simulink model "ft33_project2"  (R2024a)
settings: Solver=VariableStepAuto  StartTime=0.0  StopTime=10.0  RelTol=1e-3
undefined symbols (not defined in the file or in its folder): ft33_project2_copy, Subsystem16, xc7z020clg484
libraries: hdlBasic x111, vmcUtilities x1
(part 2 of 2)

== system ft33_project2/Subsystem16/Subsystem4 ==
  InA : Inport
  ShiftIn : Inport  Port=2
  Select : Inport  Port=3
  InB : Inport  Port=4
  Reset : Inport  Port=5
  Accumulator : hdlBasic/Accumulator  operation=Add  n_bits=16  overflow=Flag as error  scale=1  rst=on  hasbypass=off  en=off  latency=1  msb_inp=100  msb=100  lsb=-100  use_behavioral_HDL=on  implementation=Fabric  XmcBlockStatus=1  maskContainerNames=group3  block_type=accum  block_config=sysgen:Accum_config  block_width=566  block_height=845
  Delay : hdlBasic/Delay  rst=off  en=off  latency=1  reg_retiming=off  XmcBlockStatus=1  maskContainerNames=group1  block_type=delay  block_config=sysgen:Delay_config
  DelayA : hdlBasic/Register  init=0  rst=off  en=off  XmcBlockStatus=1  maskContainerNames=tabcontainer1  block_type=register  block_config=sysgen:Register_config
  DelayB : hdlBasic/Register  init=0  rst=off  en=off  XmcBlockStatus=1  maskContainerNames=tabcontainer1  block_type=register  block_config=sysgen:Register_config
  Mult : hdlBasic/Mult  precision=User Defined  arith_type="Signed  (2's comp)"  n_bits=16  bin_pt=0  quantization=Truncate  overflow=Wrap  en=off  latency=1  opt_float=off  fp_mult_usage=No Usage  use_behavioral_HDL=off  opt=Speed  use_embedded=on  optimum_pipeline=off  pipeline=on  use_rpm=on  placement_style=Triangular  XmcBlockStatus=1  maskContainerNames=group1  block_type=mult  block_config=sysgen:Mult_config  block_width=598  block_height=876
  Mux : hdlBasic/Mux  inputs=2  en=off  latency=1  precision=Full  arith_type=Unsigned  n_bits=16  bin_pt=14  quantization=Truncate  overflow=Wrap  XmcBlockStatus=1  maskContainerNames=tabcontainer1  block_type=mux  block_config=sysgen:Mux_config
  OutA : Outport
  ShiftOut : Outport  Port=2
  ResetOut : Outport  Port=3
  OutB : Outport  Port=4
  wires:
  Accumulator/1 -> Mux/2
  Mult/1 -> Accumulator/1
  InB/1 -> DelayB/1, Mult/2
  Select/1 -> Mux/1
  ShiftIn/1 -> Mux/3
  Mux/1 -> ShiftOut/1
  Reset/1 -> Delay/1, Accumulator/2
  InA/1 -> Mult/1, DelayA/1
  DelayA/1 -> OutA/1
  DelayB/1 -> OutB/1
  Delay/1 -> ResetOut/1

== system ft33_project2/Subsystem16/Subsystem5 ==
  InA : Inport
  ShiftIn : Inport  Port=2
  Select : Inport  Port=3
  InB : Inport  Port=4
  Reset : Inport  Port=5
  Accumulator : hdlBasic/Accumulator  operation=Add  n_bits=16  overflow=Flag as error  scale=1  rst=on  hasbypass=off  en=off  latency=1  msb_inp=100  msb=100  lsb=-100  use_behavioral_HDL=on  implementation=Fabric  XmcBlockStatus=1  maskContainerNames=group3  block_type=accum  block_config=sysgen:Accum_config  block_width=566  block_height=845
  Delay : hdlBasic/Delay  rst=off  en=off  latency=1  reg_retiming=off  XmcBlockStatus=1  maskContainerNames=group1  block_type=delay  block_config=sysgen:Delay_config
  DelayA : hdlBasic/Register  init=0  rst=off  en=off  XmcBlockStatus=1  maskContainerNames=tabcontainer1  block_type=register  block_config=sysgen:Register_config
  DelayB : hdlBasic/Register  init=0  rst=off  en=off  XmcBlockStatus=1  maskContainerNames=tabcontainer1  block_type=register  block_config=sysgen:Register_config
  Mult : hdlBasic/Mult  precision=User Defined  arith_type="Signed  (2's comp)"  n_bits=16  bin_pt=0  quantization=Truncate  overflow=Wrap  en=off  latency=1  opt_float=off  fp_mult_usage=No Usage  use_behavioral_HDL=off  opt=Speed  use_embedded=on  optimum_pipeline=off  pipeline=on  use_rpm=on  placement_style=Triangular  XmcBlockStatus=1  maskContainerNames=group1  block_type=mult  block_config=sysgen:Mult_config  block_width=598  block_height=876
  Mux : hdlBasic/Mux  inputs=2  en=off  latency=1  precision=Full  arith_type=Unsigned  n_bits=16  bin_pt=14  quantization=Truncate  overflow=Wrap  XmcBlockStatus=1  maskContainerNames=tabcontainer1  block_type=mux  block_config=sysgen:Mux_config
  OutA : Outport
  ShiftOut : Outport  Port=2
  ResetOut : Outport  Port=3
  OutB : Outport  Port=4
  wires:
  Accumulator/1 -> Mux/2
  Mult/1 -> Accumulator/1
  InB/1 -> DelayB/1, Mult/2
  Select/1 -> Mux/1
  ShiftIn/1 -> Mux/3
  Mux/1 -> ShiftOut/1
  Reset/1 -> Delay/1, Accumulator/2
  InA/1 -> Mult/1, DelayA/1
  DelayA/1 -> OutA/1
  DelayB/1 -> OutB/1
  Delay/1 -> ResetOut/1

== system ft33_project2/Subsystem16/Subsystem6 ==
  InA : Inport
  ShiftIn : Inport  Port=2
  ResetIn : Inport  Port=3
  Select : Inport  Port=4
  InB : Inport  Port=5
  Accumulator : hdlBasic/Accumulator  operation=Add  n_bits=16  overflow=Flag as error  scale=1  rst=on  hasbypass=off  en=off  latency=1  msb_inp=100  msb=100  lsb=-100  use_behavioral_HDL=on  implementation=Fabric  XmcBlockStatus=1  maskContainerNames=group3  block_type=accum  block_config=sysgen:Accum_config  block_width=566  block_height=845
  Delay : hdlBasic/Delay  rst=off  en=off  latency=1  reg_retiming=off  XmcBlockStatus=1  maskContainerNames=group1  block_type=delay  block_config=sysgen:Delay_config
  DelayA : hdlBasic/Register  init=0  rst=off  en=off  XmcBlockStatus=1  maskContainerNames=tabcontainer1  block_type=register  block_config=sysgen:Register_config
  DelayB : hdlBasic/Register  init=0  rst=off  en=off  XmcBlockStatus=1  maskContainerNames=tabcontainer1  block_type=register  block_config=sysgen:Register_config
  Mult : hdlBasic/Mult  precision=User Defined  arith_type="Signed  (2's comp)"  n_bits=16  bin_pt=0  quantization=Truncate  overflow=Wrap  en=off  latency=1  opt_float=off  fp_mult_usage=No Usage  use_behavioral_HDL=off  opt=Speed  use_embedded=on  optimum_pipeline=off  pipeline=on  use_rpm=on  placement_style=Triangular  XmcBlockStatus=1  maskContainerNames=group1  block_type=mult  block_config=sysgen:Mult_config  block_width=598  block_height=876
  Mux : hdlBasic/Mux  inputs=2  en=off  latency=1  precision=Full  arith_type=Unsigned  n_bits=16  bin_pt=14  quantization=Truncate  overflow=Wrap  XmcBlockStatus=1  maskContainerNames=tabcontainer1  block_type=mux  block_config=sysgen:Mux_config
  OutA : Outport
  ShiftOut : Outport  Port=2
  ResetOut : Outport  Port=3
  OutB : Outport  Port=4
  wires:
  Accumulator/1 -> Mux/2
  Mult/1 -> Accumulator/1
  InB/1 -> DelayB/1, Mult/2
  Select/1 -> Mux/1
  ShiftIn/1 -> Mux/3
  Mux/1 -> ShiftOut/1
  ResetIn/1 -> Delay/1, Accumulator/2
  InA/1 -> Mult/1, DelayA/1
  DelayA/1 -> OutA/1
  DelayB/1 -> OutB/1
  Delay/1 -> ResetOut/1

== system ft33_project2/Subsystem16/Subsystem7 ==
  InA : Inport
  ShiftIn : Inport  Port=2
  ResetIn : Inport  Port=3
  Select : Inport  Port=4
  InB : Inport  Port=5
  Accumulator : hdlBasic/Accumulator  operation=Add  n_bits=16  overflow=Flag as error  scale=1  rst=on  hasbypass=off  en=off  latency=1  msb_inp=100  msb=100  lsb=-100  use_behavioral_HDL=on  implementation=Fabric  XmcBlockStatus=1  maskContainerNames=group3  block_type=accum  block_config=sysgen:Accum_config  block_width=566  block_height=845
  Delay : hdlBasic/Delay  rst=off  en=off  latency=1  reg_retiming=off  XmcBlockStatus=1  maskContainerNames=group1  block_type=delay  block_config=sysgen:Delay_config
  DelayA : hdlBasic/Register  init=0  rst=off  en=off  XmcBlockStatus=1  maskContainerNames=tabcontainer1  block_type=register  block_config=sysgen:Register_config
  DelayB : hdlBasic/Register  init=0  rst=off  en=off  XmcBlockStatus=1  maskContainerNames=tabcontainer1  block_type=register  block_config=sysgen:Register_config
  Mult : hdlBasic/Mult  precision=User Defined  arith_type="Signed  (2's comp)"  n_bits=16  bin_pt=0  quantization=Truncate  overflow=Wrap  en=off  latency=1  opt_float=off  fp_mult_usage=No Usage  use_behavioral_HDL=off  opt=Speed  use_embedded=on  optimum_pipeline=off  pipeline=on  use_rpm=on  placement_style=Triangular  XmcBlockStatus=1  maskContainerNames=group1  block_type=mult  block_config=sysgen:Mult_config  block_width=598  block_height=876
  Mux : hdlBasic/Mux  inputs=2  en=off  latency=1  precision=Full  arith_type=Unsigned  n_bits=16  bin_pt=14  quantization=Truncate  overflow=Wrap  XmcBlockStatus=1  maskContainerNames=tabcontainer1  block_type=mux  block_config=sysgen:Mux_config
  OutA : Outport
  ShiftOut : Outport  Port=2
  ResetOut : Outport  Port=3
  OutB : Outport  Port=4
  wires:
  Accumulator/1 -> Mux/2
  Mult/1 -> Accumulator/1
  InB/1 -> DelayB/1, Mult/2
  Select/1 -> Mux/1
  ShiftIn/1 -> Mux/3
  Mux/1 -> ShiftOut/1
  ResetIn/1 -> Delay/1, Accumulator/2
  InA/1 -> Mult/1, DelayA/1
  DelayA/1 -> OutA/1
  DelayB/1 -> OutB/1
  Delay/1 -> ResetOut/1

== system ft33_project2/Subsystem16/Subsystem8 ==
  InA : Inport
  ShiftIn : Inport  Port=2
  ResetIn : Inport  Port=3
  Select : Inport  Port=4
  InB : Inport  Port=5
  Accumulator : hdlBasic/Accumulator  operation=Add  n_bits=16  overflow=Flag as error  scale=1  rst=on  hasbypass=off  en=off  latency=1  msb_inp=100  msb=100  lsb=-100  use_behavioral_HDL=on  implementation=Fabric  XmcBlockStatus=1  maskContainerNames=group3  block_type=accum  block_config=sysgen:Accum_config  block_width=566  block_height=845
  Delay : hdlBasic/Delay  rst=off  en=off  latency=1  reg_retiming=off  XmcBlockStatus=1  maskContainerNames=group1  block_type=delay  block_config=sysgen:Delay_config
  DelayA : hdlBasic/Register  init=0  rst=off  en=off  XmcBlockStatus=1  maskContainerNames=tabcontainer1  block_type=register  block_config=sysgen:Register_config
  DelayB : hdlBasic/Register  init=0  rst=off  en=off  XmcBlockStatus=1  maskContainerNames=tabcontainer1  block_type=register  block_config=sysgen:Register_config
  Mult : hdlBasic/Mult  precision=User Defined  arith_type="Signed  (2's comp)"  n_bits=16  bin_pt=0  quantization=Truncate  overflow=Wrap  en=off  latency=1  opt_float=off  fp_mult_usage=No Usage  use_behavioral_HDL=off  opt=Speed  use_embedded=on  optimum_pipeline=off  pipeline=on  use_rpm=on  placement_style=Triangular  XmcBlockStatus=1  maskContainerNames=group1  block_type=mult  block_config=sysgen:Mult_config  block_width=598  block_height=876
  Mux : hdlBasic/Mux  inputs=2  en=off  latency=1  precision=Full  arith_type=Unsigned  n_bits=16  bin_pt=14  quantization=Truncate  overflow=Wrap  XmcBlockStatus=1  maskContainerNames=tabcontainer1  block_type=mux  block_config=sysgen:Mux_config
  OutA : Outport
  ShiftOut : Outport  Port=2
  ResetOut : Outport  Port=3
  OutB : Outport  Port=4
  wires:
  Accumulator/1 -> Mux/2
  Mult/1 -> Accumulator/1
  InB/1 -> DelayB/1, Mult/2
  Select/1 -> Mux/1
  ShiftIn/1 -> Mux/3
  Mux/1 -> ShiftOut/1
  ResetIn/1 -> Delay/1, Accumulator/2
  InA/1 -> Mult/1, DelayA/1
  DelayA/1 -> OutA/1
  DelayB/1 -> OutB/1
  Delay/1 -> ResetOut/1

== system ft33_project2/Subsystem16/Subsystem9 ==
  InA : Inport
  ShiftIn : Inport  Port=2
  ResetIn : Inport  Port=3
  Select : Inport  Port=4
  InB : Inport  Port=5
  Accumulator : hdlBasic/Accumulator  operation=Add  n_bits=16  overflow=Flag as error  scale=1  rst=on  hasbypass=off  en=off  latency=1  msb_inp=100  msb=100  lsb=-100  use_behavioral_HDL=on  implementation=Fabric  XmcBlockStatus=1  maskContainerNames=group3  block_type=accum  block_config=sysgen:Accum_config  block_width=566  block_height=845
  Delay : hdlBasic/Delay  rst=off  en=off  latency=1  reg_retiming=off  XmcBlockStatus=1  maskContainerNames=group1  block_type=delay  block_config=sysgen:Delay_config
  DelayA : hdlBasic/Register  init=0  rst=off  en=off  XmcBlockStatus=1  maskContainerNames=tabcontainer1  block_type=register  block_config=sysgen:Register_config
  DelayB : hdlBasic/Register  init=0  rst=off  en=off  XmcBlockStatus=1  maskContainerNames=tabcontainer1  block_type=register  block_config=sysgen:Register_config
  Mult : hdlBasic/Mult  precision=User Defined  arith_type="Signed  (2's comp)"  n_bits=16  bin_pt=0  quantization=Truncate  overflow=Wrap  en=off  latency=1  opt_float=off  fp_mult_usage=No Usage  use_behavioral_HDL=off  opt=Speed  use_embedded=on  optimum_pipeline=off  pipeline=on  use_rpm=on  placement_style=Triangular  XmcBlockStatus=1  maskContainerNames=group1  block_type=mult  block_config=sysgen:Mult_config  block_width=598  block_height=876
  Mux : hdlBasic/Mux  inputs=2  en=off  latency=1  precision=Full  arith_type=Unsigned  n_bits=16  bin_pt=14  quantization=Truncate  overflow=Wrap  XmcBlockStatus=1  maskContainerNames=tabcontainer1  block_type=mux  block_config=sysgen:Mux_config
  OutA : Outport
  ShiftOut : Outport  Port=2
  ResetOut : Outport  Port=3
  OutB : Outport  Port=4
  wires:
  Accumulator/1 -> Mux/2
  Mult/1 -> Accumulator/1
  InB/1 -> DelayB/1, Mult/2
  Select/1 -> Mux/1
  ShiftIn/1 -> Mux/3
  Mux/1 -> ShiftOut/1
  ResetIn/1 -> Delay/1, Accumulator/2
  InA/1 -> Mult/1, DelayA/1
  DelayA/1 -> OutA/1
  DelayB/1 -> OutB/1
  Delay/1 -> ResetOut/1
